simulink model "Anti_windup_slk"  (R2023b)
settings: Solver=VariableStepAuto  StartTime=0.0  StopTime=Tend_slk  RelTol=1e-3
values from neighbouring files (symbols this model uses):
  A_cond = A-B*inv(D)*C    [Anti_windup.m]
  B_cond = B*inv(D)    [Anti_windup.m]
  C = R_final_ss.C    [Anti_windup.m]
  D = R_final_ss.D    [Anti_windup.m]
  K = [-0.17658959407 -0.180363931417]    [K_H2_1dof_new_Ixx.mat]
  param = [Ixx;Iyy;Izz;l;k1;k2;k3;k4;b;m]    [Anti_windup.m]
  tau_r = 0.01    [Anti_windup.m]
  Ts_slk = 0.001    [Anti_windup.m]
  x0 = [0;0]    [Anti_windup.m]
libraries: cstblocks x9, simulink x6, slpidlib x2
settings Model: Creator=asus  LastModifiedBy=asus

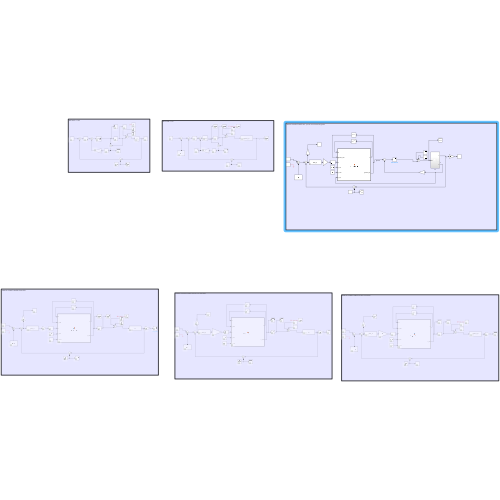
[thumbnail: Simulink's stored preview of the top-level diagram]
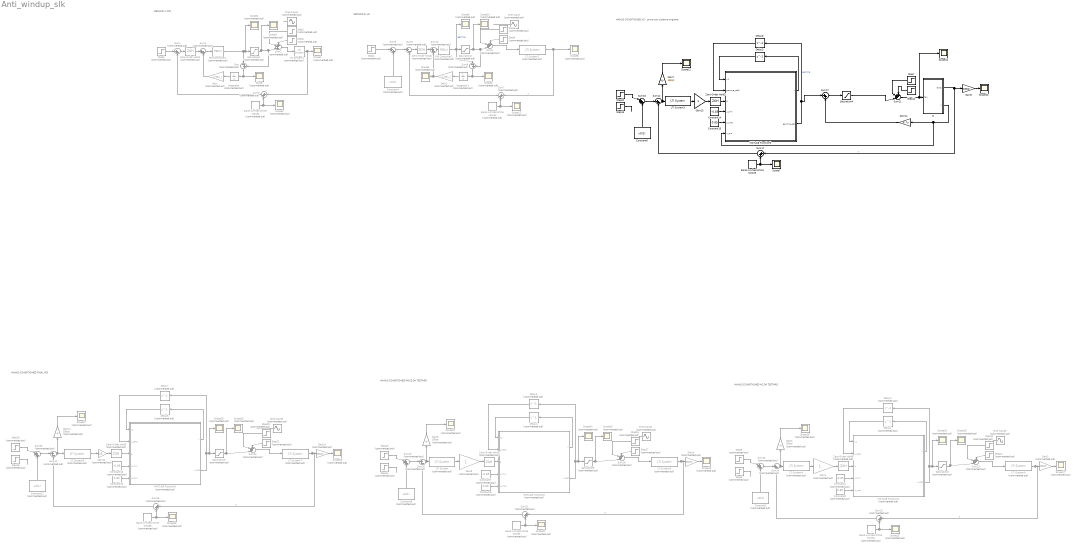
== system Anti_windup_slk ==
  note: METHOD 1: PID
  note: METHOD 3: H2
  note: HANUS CONDITIONED POLE DA TESTARE
  note: HANUS CONDITIONED FINAL PID
  note: HANUS CONDITIONED H2 DA TESTARE
  note: HANUS CONDITIONED H2 - prova con sistema originale
  Band-Limited White Noise{1..2,4..6} (5 alike) : simulink/Sources/Band-Limited White Noise  Commented=on  Cov=[0.0001]  Ts=0.05  seed=[23341]
  Band-Limited White Noise3 : simulink/Sources/Band-Limited White Noise  Cov=[0.0001]  Ts=0.05  seed=[23341]
  Constant1 : Constant  Commented=on  Value=-0.85  SampleTime=Ts_slk
  Constant10 : Constant  Commented=on  Value=-0.85  SampleTime=Ts_slk
  Constant{2,4,8,11} (4 alike) : Constant  Commented=on  Value=x0(1)
  Constant12 : Constant  Commented=on  Value=0.85  SampleTime=Ts_slk
  Constant14 : Constant  Value=-0.85  SampleTime=Ts_slk
  Constant15 : Constant  Value=0.85  SampleTime=Ts_slk
  Constant5 : Constant  Commented=on  Value=0.85  SampleTime=Ts_slk
  Constant6 : Constant  Value=x0(1)
  Constant7 : Constant  Commented=on  Value=-0.85  SampleTime=Ts_slk
  Constant9 : Constant  Commented=on  Value=0.85  SampleTime=Ts_slk
  Delay1 : Delay  Commented=on  DelayLength=1  InitialCondition=zeros(5,1)  SampleTime=Ts_slk
  Delay2 : Delay  Commented=on  DelayLength=1  InitialCondition=0  SampleTime=Ts_slk
  Delay3 : Delay  DelayLength=1  InitialCondition=zeros(5,1)  SampleTime=Ts_slk
  Delay4 : Delay  Commented=on  DelayLength=1  InitialCondition=zeros(3,1)  SampleTime=Ts_slk
  Delay5 : Delay  Commented=on  DelayLength=1  InitialCondition=0  SampleTime=Ts_slk
  Delay6 : Delay  Commented=on  DelayLength=1  InitialCondition=zeros(2,1)  SampleTime=Ts_slk
  Delay7 : Delay  Commented=on  DelayLength=1  InitialCondition=0  SampleTime=Ts_slk
  Delay8 : Delay  DelayLength=1  InitialCondition=0  SampleTime=Ts_slk
  G : Subsystem
  Gain : Gain  Commented=on  Gain=1/tau_r
  Gain1 : Gain  Commented=on  Gain=1/tau_r
  Gain{2..3,5,8,10..11} (6 alike) : Gain  Commented=on  Gain=180/pi
  Gain12 : Gain  Commented=on  Gain=35
  Gain13 : Gain
  Gain14 : Gain  Gain=K  Multiplication=Matrix(K*u)
  Gain4 : Gain  Commented=on
  Gain6 : Gain  Gain=180/pi
  Gain7 : Gain  Gain=180/pi
  Gain9 : Gain  Commented=on
  Integrator : Integrator  Commented=on
  Integrator1 : Integrator  Commented=on
  LTI System : cstblocks/LTI System  Commented=on  sys=filter_d  IC=[]  PadeOrder=0
  LTI System1 : cstblocks/LTI System  Commented=on  sys=G  IC=[]  PadeOrder=0
  LTI System2 : cstblocks/LTI System  Commented=on  sys=stable_sys  IC=[]  PadeOrder=0
  LTI System3 : cstblocks/LTI System  sys=filter_d  IC=[]  PadeOrder=0
  LTI System4 : cstblocks/LTI System  Commented=on  sys=filter_d  IC=[]  PadeOrder=0
  LTI System5 : cstblocks/LTI System  Commented=on  sys=G  IC=[]  PadeOrder=0
  LTI System6 : cstblocks/LTI System  Commented=on  sys=filter_d  IC=[]  PadeOrder=0
  LTI System7 : cstblocks/LTI System  Commented=on  sys=G  IC=[]  PadeOrder=0
  LTI System9 : cstblocks/LTI System  Commented=on  sys=stable_sys  IC=[]  PadeOrder=0
  MATLAB Function1 : MATLAB Function  Commented=on  TreatAsAtomicUnit=on
  MATLAB Function2 : MATLAB Function  Commented=on  TreatAsAtomicUnit=on
  MATLAB Function3 : MATLAB Function  Commented=on  TreatAsAtomicUnit=on
  MATLAB Function5 : MATLAB Function  TreatAsAtomicUnit=on
  PID Controller1 : slpidlib/PID Controller  Commented=on  Controller=PID  Form=Parallel  TimeDomain=Continuous-time  UseExternalTs=off  SampleTime=Ts_slk  IntegratorMethod=Forward Euler  FilterMethod=Forward Euler  ControllerParametersSource=internal  P=0.0408494379196507*4  I=0.00382471475812365  UseKiTs=off  D=0.107131307975801  N=10.9079405084324  UseFilter=on  TunerSelectOption=Transfer Function Based (PID Tuner App)  InitialConditionSource=internal  InitialConditionForIntegrator=0  InitialConditionForFilter=0  DifferentiatorICPrevScaledInput=0  ExternalReset=none  TrackingMode=off  Kt=1  LimitOutput=on  SatLimitsSource=internal  UpperSaturationLimit=1.2  LowerSaturationLimit=-1.2  LinearizeAsGain=on  AntiWindupMode=clamping  Kb=1  LimitIntegrator=off  UpperIntegratorSaturationLimit=inf  LowerIntegratorSaturationLimit=-inf  POutMin=[]  POutMax=[]  IOutMin=[]  IOutMax=[]  DOutMin=[]  DOutMax=[]  NOutMin=[]  NOutMax=[]  SumOutMin=[]  SumOutMax=[]  SaturationOutMin=[]  SaturationOutMax=[]  PParamMin=[]  PParamMax=[]  IParamMin=[]  IParamMax=[]  DParamMin=[]  DParamMax=[]  NParamMin=[]  NParamMax=[]  KbParamMin=[]  KbParamMax=[]  KtParamMin=[]  KtParamMax=[]  KbOutMin=[]  KbOutMax=[]  KtOutMin=[]  KtOutMax=[]  IntegratorOutMin=[]  IntegratorOutMax=[]  FilterOutMin=[]  FilterOutMax=[]  SumI1OutMin=[]  SumI1OutMax=[]  SumI2OutMin=[]  SumI2OutMax=[]  SumI3OutMin=[]  SumI3OutMax=[]  SumI4OutMin=[]  SumI4OutMax=[]  SumDOutMin=[]  SumDOutMax=[]  DifferentiatorOutMin=[]  DifferentiatorOutMax=[]  FilterDiffOutCoefMin=[]  FilterDiffOutCoefMax=[]  ReciprocalOutMin=[]  ReciprocalOutMax=[]  SumDenOutMin=[]  SumDenOutMax=[]  SumNumOutMin=[]  SumNumOutMax=[]  DivideOutMin=[]  DivideOutMax=[]  UdiffTsProdOutMin=[]  UdiffTsProdOutMax=[]  NTsProdOutMin=[]  NTsProdOutMax=[]  UintegralTsProdOutMin=[]  UintegralTsProdOutMax=[]  UngainTsProdOutMin=[]  UngainTsProdOutMax=[]  ClampingZeroOutDataTypeStr=Inherit: Inherit via back propagation  ClampingZeroOutMin=[]  ClampingZeroOutMax=[]  FilterDenConstantOutDataTypeStr=Inherit: Inherit via back propagation  FilterDenConstantOutMin=[]  FilterDenConstantOutMax=[]  PCopyOutDataTypeStr=Inherit: Inherit via back propagation  PCopyOutMin=[]  PCopyOutMax=[]  NCopyOutDataTypeStr=Inherit: Inherit via back propagation  NCopyOutMin=[]  NCopyOutMax=[]  IntegratorContinuousStateAttributes=''  IntegratorStateMustResolveToSignalObject=off  IntegratorRTWStateStorageClass=Auto  FilterContinuousStateAttributes=''  FilterStateMustResolveToSignalObject=off  FilterRTWStateStorageClass=Auto  ParallelPVariant=InternalParameters  IdealPVariant=Disabled  IVariant=InternalParameters  DVariant=InternalParameters  IntegratorVariant=Continuous  SatVariant=Enabled  AWVariant=ContClampingParallel  PCopyVariant=Disabled  TRVariant=Disabled  FdbkBlocksVariant=Forward  IdealPFdbkVariant=Disabled  SatFdbkVariant=Disabled  DerivativeFilterVariant=ContFilter  NVariant=InternalParameters  NCopyVariant=Disabled  FilterICVariant=InternalICsFilter  IntegratorICVariant=InternalICs  ExternalResetVariant=Disabled  TRSumVariant=Passthrough  SumFdbkVariant=Disabled  SumVariant=Sum_PID  TsampFilterVariant=InternalTs  TsampNgainVariant=Passthrough  TsampIntegralVariant=Disabled_SignalSpec  ExternalSaturationOutDataTypeStr=Inherit: Same as second input
  PID Controller2 : slpidlib/PID Controller  Commented=on  Controller=PID  Form=Parallel  TimeDomain=Continuous-time  UseExternalTs=off  SampleTime=Ts_slk  IntegratorMethod=Forward Euler  FilterMethod=Forward Euler  ControllerParametersSource=internal  P=0.358963618588833  I=0.316424724366205  UseKiTs=off  D=0.100819102821921  N=228.565595208321  UseFilter=on  TunerSelectOption=Transfer Function Based (PID Tuner App)  InitialConditionSource=internal  InitialConditionForIntegrator=0  InitialConditionForFilter=0  DifferentiatorICPrevScaledInput=0  ExternalReset=none  TrackingMode=off  Kt=1  LimitOutput=off  SatLimitsSource=internal  UpperSaturationLimit=1.2  LowerSaturationLimit=-1.2  LinearizeAsGain=on  AntiWindupMode=clamping  Kb=1  LimitIntegrator=off  UpperIntegratorSaturationLimit=inf  LowerIntegratorSaturationLimit=-inf  POutMin=[]  POutMax=[]  IOutMin=[]  IOutMax=[]  DOutMin=[]  DOutMax=[]  NOutMin=[]  NOutMax=[]  SumOutMin=[]  SumOutMax=[]  SaturationOutMin=[]  SaturationOutMax=[]  PParamMin=[]  PParamMax=[]  IParamMin=[]  IParamMax=[]  DParamMin=[]  DParamMax=[]  NParamMin=[]  NParamMax=[]  KbParamMin=[]  KbParamMax=[]  KtParamMin=[]  KtParamMax=[]  KbOutMin=[]  KbOutMax=[]  KtOutMin=[]  KtOutMax=[]  IntegratorOutMin=[]  IntegratorOutMax=[]  FilterOutMin=[]  FilterOutMax=[]  SumI1OutMin=[]  SumI1OutMax=[]  SumI2OutMin=[]  SumI2OutMax=[]  SumI3OutMin=[]  SumI3OutMax=[]  SumI4OutMin=[]  SumI4OutMax=[]  SumDOutMin=[]  SumDOutMax=[]  DifferentiatorOutMin=[]  DifferentiatorOutMax=[]  FilterDiffOutCoefMin=[]  FilterDiffOutCoefMax=[]  ReciprocalOutMin=[]  ReciprocalOutMax=[]  SumDenOutMin=[]  SumDenOutMax=[]  SumNumOutMin=[]  SumNumOutMax=[]  DivideOutMin=[]  DivideOutMax=[]  UdiffTsProdOutMin=[]  UdiffTsProdOutMax=[]  NTsProdOutMin=[]  NTsProdOutMax=[]  UintegralTsProdOutMin=[]  UintegralTsProdOutMax=[]  UngainTsProdOutMin=[]  UngainTsProdOutMax=[]  ClampingZeroOutDataTypeStr=Inherit: Inherit via back propagation  ClampingZeroOutMin=[]  ClampingZeroOutMax=[]  FilterDenConstantOutDataTypeStr=Inherit: Inherit via back propagation  FilterDenConstantOutMin=[]  FilterDenConstantOutMax=[]  PCopyOutDataTypeStr=Inherit: Inherit via back propagation  PCopyOutMin=[]  PCopyOutMax=[]  NCopyOutDataTypeStr=Inherit: Inherit via back propagation  NCopyOutMin=[]  NCopyOutMax=[]  IntegratorContinuousStateAttributes=''  IntegratorStateMustResolveToSignalObject=off  IntegratorRTWStateStorageClass=Auto  FilterContinuousStateAttributes=''  FilterStateMustResolveToSignalObject=off  FilterRTWStateStorageClass=Auto  ParallelPVariant=InternalParameters  IdealPVariant=Disabled  IVariant=InternalParameters  DVariant=InternalParameters  IntegratorVariant=Continuous  SatVariant=Disabled  AWVariant=Passthrough  PCopyVariant=Disabled  TRVariant=Disabled  FdbkBlocksVariant=Forward  IdealPFdbkVariant=Disabled  SatFdbkVariant=Disabled  DerivativeFilterVariant=ContFilter  NVariant=InternalParameters  NCopyVariant=Disabled  FilterICVariant=InternalICsFilter  IntegratorICVariant=InternalICs  ExternalResetVariant=Disabled  TRSumVariant=Passthrough  SumFdbkVariant=Disabled  SumVariant=Sum_PID  TsampFilterVariant=InternalTs  TsampNgainVariant=Passthrough  TsampIntegralVariant=Disabled_SignalSpec  ExternalSaturationOutDataTypeStr=Inherit: Same as second input
  Saturation1 : Saturate  Commented=on  UpperLimit=1.2  LowerLimit=-1.2
  Saturation2 : Saturate  Commented=on  UpperLimit=1.2  LowerLimit=-1.2
  Saturation3 : Saturate  Commented=on  UpperLimit=0.85  LowerLimit=-0.85
  Saturation4 : Saturate  UpperLimit=0.85  LowerLimit=-0.85
  Saturation5 : Saturate  Commented=on  UpperLimit=0.85  LowerLimit=-0.85
  Saturation6 : Saturate  Commented=on  UpperLimit=0.85  LowerLimit=-0.85
  Scope{,1..6,8..11,15..19,21..30} (26 alike) : Scope  Commented=on
  Scope{7,12..14} (4 alike) : Scope
  Sine Wave{,3..5} (4 alike) : Sin  Commented=on  Amplitude=0.2  Frequency=4  SampleTime=Ts_slk
  Sine Wave1 : Sin  Commented=on  Amplitude=0.2  Frequency=5  SampleTime=Ts_slk
  Step{1,5,10,16,20} (5 alike) : Step  Commented=on  Time=100  After=0.2  SampleTime=Ts_slk
  Step{2,6,11,17,21} (5 alike) : Step  Commented=on  Time=100.1  After=-0.2  SampleTime=Ts_slk
  Step12 : Step  Time=100.1  After=-0.2  SampleTime=Ts_slk
  Step13 : Step  Time=50  After=-0.52  SampleTime=Ts_slk
  Step14 : Step  Commented=on  Time=50  After=-0.52  SampleTime=Ts_slk
  Step{3,9,15,19} (4 alike) : Step  Commented=on  Time=0  After=0.5  SampleTime=Ts_slk
  Step18 : Step  Commented=on  Time=50  After=-0.52  SampleTime=Ts_slk
  Step22 : Step  Time=0  After=0.5  SampleTime=Ts_slk
  Step4 : Step  Commented=on  Time=0  After=0.52  SampleTime=Ts_slk
  Step7 : Step  Time=100  After=0.2  SampleTime=Ts_slk
  Step8 : Step  Commented=on  Time=50  After=-0.52  SampleTime=Ts_slk
  Sum : Sum  Commented=on  Inputs=|-+
  Sum{1,6,14,20,24} (5 alike) : Sum  Commented=on  Inputs=|+-
  Sum{3..4,7,9..10,15,21,25} (8 alike) : Sum  Commented=on  Inputs=|++
  Sum11 : Sum  Inputs=+++|
  Sum12 : Sum  Inputs=|+-
  Sum{2,5,13,19,23} (5 alike) : Sum  Commented=on  Inputs=+++|
  Sum16 : Sum  Commented=on  Inputs=|+++
  Sum17 : Sum  Inputs=|++
  Sum18 : Sum  Inputs=|+++
  Sum22 : Sum  Commented=on  Inputs=|+++
  Sum26 : Sum  Commented=on  Inputs=|+++
  Sum27 : Sum  Inputs=|++
  Sum8 : Sum  Commented=on  Inputs=|-+
  Zero-Order Hold{1..2,4..6} (5 alike) : ZeroOrderHold  Commented=on  SampleTime=Ts_slk
  Zero-Order Hold3 : ZeroOrderHold  SampleTime=Ts_slk
  wires:
  Sine Wave1/1 -> ?
  Sum3/1 -> Sum1/2
  Step3/1 -> Sum1/1
  Step1/1 -> Sum2/2
  Saturation1/1 -> Scope3/1, Sum/2, Sum2/3
  Sum2/1 -> LTI System1/1
  LTI System1/1 -> Sum3/1, Scope1/1
  Sum1/1 -> Zero-Order Hold1/1
  Step2/1 -> Sum2/1
  Band-Limited White Noise1/1 -> Scope4/1, Sum3/2
  PID Controller1/1 -> Sum/1, Saturation1/1, Scope2/1
  Zero-Order Hold1/1 -> Sum4/1
  Gain/1 -> Sum4/2
  Sum4/1 -> PID Controller1/1
  Integrator/1 -> Gain/1
  Sum/1 -> Integrator/1, Scope/1
  Sine Wave/1 -> ?
  Step6/1 -> Sum5/1
  Step4/1 -> Sum9/1
  LTI System2/1 -> Sum7/1, Scope8/1  "y"
  Constant4/1 -> Sum9/2
  Band-Limited White Noise2/1 -> Scope11/1, Sum7/2
  PID Controller2/1 -> Saturation2/1, Sum8/1, Scope9/1  "gamma"
  Zero-Order Hold2/1 -> Sum10/1
  Sum7/1 -> Sum6/2
  Step5/1 -> Sum5/2
  Sum5/1 -> LTI System2/1
  Sum9/1 -> Sum6/1
  Sum6/1 -> Zero-Order Hold2/1
  Integrator1/1 -> Gain1/1
  Sum8/1 -> Integrator1/1, Scope5/1
  Gain1/1 -> Sum10/2, Scope6/1
  Saturation2/1 -> Scope10/1, Sum8/2, Sum5/3
  Sum10/1 -> PID Controller2/1
  Sine Wave4/1 -> ?
  Sum20/1 -> Gain8/1, LTI System/1
  Step14/1 -> ?
  Gain5/1 -> Scope23/1
  Step17/1 -> Sum19/1
  Constant8/1 -> Sum22/3
  Delay4/1 -> MATLAB Function2/1(x1)
  Sum19/1 -> LTI System5/1
  MATLAB Function2/2(u_sat) -> Scope24/1, Saturation5/1, Delay5/1
  Step15/1 -> Sum22/1
  Sum22/1 -> Sum20/1
  MATLAB Function2/1(x) -> Delay4/1
  Constant7/1 -> MATLAB Function2/4(u_min)
  Band-Limited White Noise5/1 -> Sum21/2, Scope21/1
  Step16/1 -> Sum19/2
  Sum21/1 -> Sum20/2
  Saturation5/1 -> Scope25/1, Sum19/3
  Delay5/1 -> MATLAB Function2/2(u_sat1)
  Gain8/1 -> Scope22/1
  LTI System5/1 -> Sum21/1, Gain5/1  "y"
  Constant9/1 -> MATLAB Function2/5(u_max)
  LTI System/1 -> Gain9/1
  Gain9/1 -> Zero-Order Hold4/1
  Zero-Order Hold4/1 -> MATLAB Function2/3(e)
  MATLAB Function3/1(x) -> Delay6/1
  Delay6/1 -> MATLAB Function3/1(x1)
  Sum26/1 -> Sum24/1
  Sum24/1 -> Gain11/1, LTI System6/1
  Gain10/1 -> Scope28/1
  Step21/1 -> Sum23/1
  Step18/1 -> ?
  Sine Wave5/1 -> ?
  LTI System7/1 -> Sum25/1, Gain10/1  "y"
  Constant12/1 -> MATLAB Function3/5(u_max)
  MATLAB Function3/2(u_sat) -> Scope29/1, Saturation6/1, Delay7/1
  Sum23/1 -> LTI System7/1
  Constant10/1 -> MATLAB Function3/4(u_min)
  Band-Limited White Noise6/1 -> Sum25/2, Scope26/1
  Zero-Order Hold5/1 -> MATLAB Function3/3(e)
  Constant11/1 -> Sum26/3
  Gain11/1 -> Scope27/1
  Step20/1 -> Sum23/2
  Sum25/1 -> Sum24/2
  Saturation6/1 -> Scope30/1, Sum23/3
  LTI System6/1 -> Gain12/1
  Delay7/1 -> MATLAB Function3/2(u_sat1)
  Gain12/1 -> Zero-Order Hold5/1
  Step19/1 -> Sum26/1
  Step8/1 -> ?
  Sum15/1 -> Sum14/2
  Delay1/1 -> MATLAB Function1/1(x1)
  Delay2/1 -> MATLAB Function1/2(u_sat1)
  MATLAB Function1/2(u_sat) -> Scope18/1, Saturation3/1, Delay2/1
  LTI System9/1 -> Sum15/1, Gain2/1  "y"
  Step9/1 -> Sum16/1
  Gain3/1 -> Scope16/1
  LTI System4/1 -> Gain4/1
  Saturation3/1 -> Scope19/1, Sum13/3
  Step11/1 -> Sum13/1
  Constant5/1 -> MATLAB Function1/5(u_max)
  Zero-Order Hold6/1 -> MATLAB Function1/3(e)
  Step10/1 -> Sum13/2
  Sum16/1 -> Sum14/1
  Sum13/1 -> LTI System9/1
  Gain2/1 -> Scope17/1
  Constant1/1 -> MATLAB Function1/4(u_min)
  Gain4/1 -> Zero-Order Hold6/1
  Band-Limited White Noise4/1 -> Sum15/2, Scope15/1
  Sine Wave3/1 -> ?
  MATLAB Function1/1(x) -> Delay1/1
  Constant2/1 -> Sum16/3
  Sum14/1 -> Gain3/1, LTI System4/1
  Step13/1 -> ?
  Sum12/1 -> Gain7/1, LTI System3/1
  Step22/1 -> Sum18/1
  LTI System3/1 -> Gain13/1
  Gain6/1 -> Scope13/1
  Step7/1 -> Sum11/2
  Gain7/1 -> Scope12/1
  Saturation4/1 -> Sum11/3
  Sum18/1 -> Sum12/1
  Step12/1 -> Sum11/1
  Band-Limited White Noise3/1 -> Sum17/2, Scope7/1
  Constant6/1 -> Sum18/3
  Sum17/1 -> Sum12/2
  Sum11/1 -> Scope14/1, G/1("tau ")
  G/1(Out1) -> Sum17/1, Gain6/1  "y"
  G/2(x) -> MATLAB Function5/6(x_sys), Gain14/1
  Gain14/1 -> Sum27/2
  Sum27/1 -> Saturation4/1
  Delay3/1 -> MATLAB Function5/1(x1)
  MATLAB Function5/1(x) -> Delay3/1
  Constant14/1 -> MATLAB Function5/4(u_min)
  Zero-Order Hold3/1 -> MATLAB Function5/3(e)
  MATLAB Function5/2(gamma_sat) -> Sum27/1, Delay8/1  "gamma"
  Delay8/1 -> MATLAB Function5/2(gamma_sat1)
  Constant15/1 -> MATLAB Function5/5(u_max)
  Gain13/1 -> Zero-Order Hold3/1

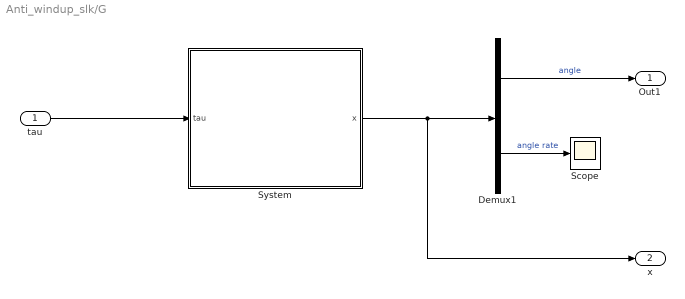
== system Anti_windup_slk/G ==
  "tau " : Inport
  Demux1 : Demux  Outputs=2
  Scope : Scope
  System : Subsystem
  Out1 : Outport
  x : Outport  Port=2
  wires:
  System/1(x) -> x/1, Demux1/1
  "tau "/1 -> System/1("tau ")
  Demux1/2 -> Scope/1  "angle rate"
  Demux1/1 -> Out1/1  "angle"

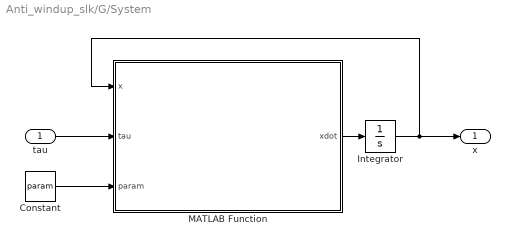
== system Anti_windup_slk/G/System ==
  "tau " : Inport
  Constant : Constant  Value=param
  Integrator : Integrator  InitialCondition=x0
  MATLAB Function : MATLAB Function  TreatAsAtomicUnit=on
  x : Outport
  wires:
  Integrator/1 -> MATLAB Function/1(x), x/1
  MATLAB Function/1(xdot) -> Integrator/1
  "tau "/1 -> MATLAB Function/2(tau)
  Constant/1 -> MATLAB Function/3(param)

== matlab function Anti_windup_slk/MATLAB Function1 ==
  data: x1 input; x output; u_sat1 input; e input; u_sat output; A_cond parameter; B_cond parameter; C parameter; D parameter; u_min input; u_max input
function [x,u_sat]= PID_controller(x1,u_sat1,e, A_cond, B_cond, C, D, u_min, u_max)
x       =   A_cond*x1 + B_cond*u_sat1;
u       =   C*x + D*e;
u_sat   =   max(u_min, min (u_max, u));

== matlab function Anti_windup_slk/MATLAB Function2 ==
  data: x1 input; x output; u_sat1 input; e input; u_sat output; A_cond parameter; B_cond parameter; C parameter; D parameter; u_min input; u_max input
function [x,u_sat]= PID_controller(x1,u_sat1,e, A_cond, B_cond, C, D, u_min, u_max)
x       =   A_cond*x1 + B_cond*u_sat1;
u       =   C*x + D*e;
u_sat   =   max(u_min, min (u_max, u));

== matlab function Anti_windup_slk/MATLAB Function3 ==
  data: x1 input; x output; u_sat1 input; e input; u_sat output; A_cond parameter; B_cond parameter; C parameter; D parameter; u_min input; u_max input
function [x,u_sat]= PID_controller(x1,u_sat1,e, A_cond, B_cond, C, D, u_min, u_max)
x       =   A_cond*x1 + B_cond*u_sat1;
u       =   C*x + D*e;
u_sat   =   max(u_min, min (u_max, u));

== matlab function Anti_windup_slk/G/System/MATLAB Function ==
  data: x input; tau input; xdot output; param input
function xdot=quadcopter(x,tau,param)
% Inputs:
%           x       (model state)
%           tau     (torque)           
%           param   (model parameters)
%
% Outputs:  x_dot  (derivative of the state with respect to time)

% Parameters
g        =       9.81;           %  gravity acceleration (m/s^2)
Ixx      =       param(1,1);     %  moment of inertia 

% States
phi         =       x(1,1);      %  roll angle (rad)
phi_dot     =       x(2,1);      %  roll rate (rad/s)


cph         =       cos(phi);
sph         =       sin(phi);

% State space model
xdot        = zeros(2,1);
xdot(1,1)   = phi_dot;
xdot(2,1)   = tau/Ixx;

== matlab function Anti_windup_slk/MATLAB Function5 ==
  data: x1 input; x output; gamma_sat1 input; e input; gamma_sat output; A_cond parameter; B_cond parameter; C parameter; D parameter; u_min input; u_max input; x_sys input; K parameter
function [x,gamma_sat]= PID_controller(x1,gamma_sat1,e, A_cond, B_cond, C, D, u_min, u_max, x_sys, K)
x           =   A_cond*x1 + B_cond*gamma_sat1;
gamma       =   C*x + D*e;
u           =   gamma + K*x_sys;
u_sat       =   max(u_min, min (u_max, u));  
gamma_sat   =   u-K*x_sys;
